simulink model "WhiteBlancing_using_difference_of_255"  (R2016a)
settings: Solver=VariableStepAuto  StartTime=0.0  StopTime=10.0  RelTol=1e-3
undefined symbols (not defined in the file): Rec, SDTV
libraries: visionsources x2, visionsinks x2, visionconversions x1
settings Model: Creator=YASARA  LastModifiedBy=YASARA

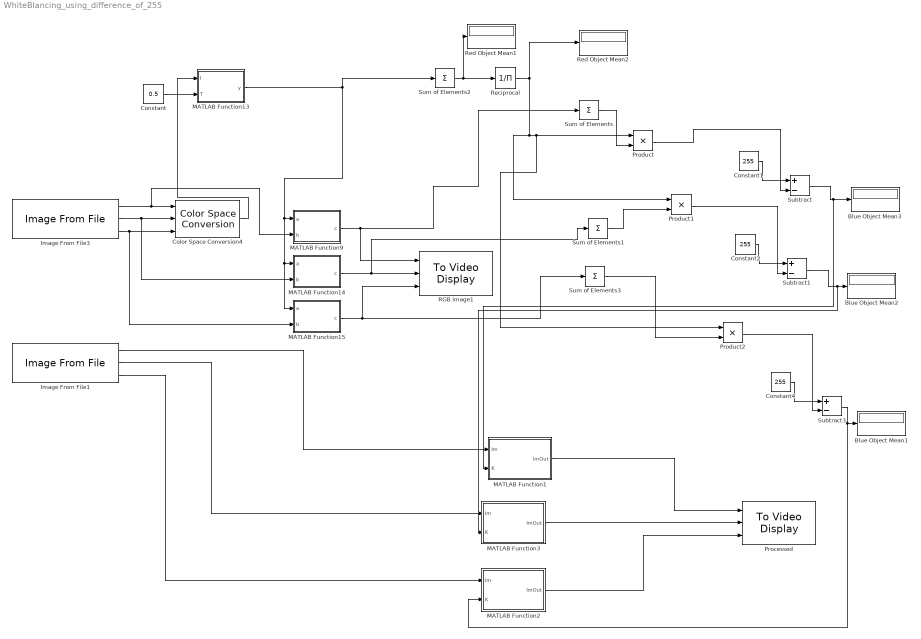
== system WhiteBlancing_using_difference_of_255 ==
  Blue Object Mean1 : Display
  Blue Object Mean2 : Display
  Blue Object Mean3 : Display
  Color Space Conversion4 : visionconversions/Color Space  Conversion  conversion=Obsolete  conversionActive=R'G'B' to intensity  wp_str=D65  rec=Rec. 601 (SDTV)  sys=1125/60/2:1  imagePorts=Separate color signals
  Constant : Constant  Value=0.5  SampleTime=1
  Constant1 : Constant  Value=255
  Constant2 : Constant  Value=255
  Constant4 : Constant  Value=255
  Image From File1 : visionsources/Image From File  Tag=vipblks_nd  FileName=C:\Users\YASARA\Desktop\FRY_Docu\tea\teaxb.jpg  imagePorts=Separate color signals  Ts=1  ImageDataType=uint8  Signed=on  WordLength=16  sdImageDataType=uint(8)  FractionLengthMode=User-defined  FractionLength=15  OutPortLabels=R|G|B
  Image From File3 : visionsources/Image From File  Tag=vipblks_nd  FileName=C:\Users\YASARA\Desktop\FRY_Docu\tea\teaxb.jpg  imagePorts=Separate color signals  Ts=1  ImageDataType=single  Signed=on  WordLength=16  sdImageDataType=uint(8)  FractionLengthMode=User-defined  FractionLength=15  OutPortLabels=R|G|B
  MATLAB Function1 : MATLAB Function  TreatAsAtomicUnit=on
  MATLAB Function13 : MATLAB Function  TreatAsAtomicUnit=on
  MATLAB Function14 : MATLAB Function  TreatAsAtomicUnit=on
  MATLAB Function15 : MATLAB Function  TreatAsAtomicUnit=on
  MATLAB Function2 : MATLAB Function  TreatAsAtomicUnit=on
  MATLAB Function3 : MATLAB Function  TreatAsAtomicUnit=on
  MATLAB Function9 : MATLAB Function  TreatAsAtomicUnit=on
  Processed : visionsinks/To Video Display  windowSizeMode=Normal  openAtMdlStart=on  fullScreen=off  videoWindowX=252  videoWindowY=213  saveWindowSize=off  videoWindowWidth=512  videoWindowHeight=384  inputColorFormat=RGB  inputType=Obsolete  imagePorts=Separate color signals  OutputDevice=On-screen video monitor  dataOrg=Column-major  isWindowOpen=off
  Product : Product  OutDataTypeStr=uint8
  Product1 : Product  OutDataTypeStr=uint8
  Product2 : Product  OutDataTypeStr=uint8
  RGB image1 : visionsinks/To Video Display  windowSizeMode=Normal  openAtMdlStart=on  fullScreen=off  videoWindowX=252  videoWindowY=213  saveWindowSize=off  videoWindowWidth=512  videoWindowHeight=384  inputColorFormat=RGB  inputType=Obsolete  imagePorts=Separate color signals  OutputDevice=On-screen video monitor  dataOrg=Column-major  isWindowOpen=off
  Reciprocal : Product  Inputs=/  OutDataTypeStr=double  SaturateOnIntegerOverflow=on  RndMeth=Zero
  Red Object Mean1 : Display
  Red Object Mean2 : Display
  Subtract : Sum  Inputs=+-
  Subtract1 : Sum  Inputs=+-
  Subtract3 : Sum  Inputs=+-
  Sum of Elements : Sum  Inputs=+
  Sum of Elements1 : Sum  Inputs=+
  Sum of Elements2 : Sum  Inputs=+  AccumDataTypeStr=uint8  OutDataTypeStr=uint8
  Sum of Elements3 : Sum  Inputs=+
  wires:
  Color Space Conversion4/1 -> MATLAB Function13/1(I)
  Sum of Elements/1 -> Product/2
  MATLAB Function9/1(c) -> RGB image1/1, Sum of Elements/1
  MATLAB Function14/1(c) -> RGB image1/2, Sum of Elements1/1
  Sum of Elements3/1 -> Product2/2
  MATLAB Function15/1(c) -> Sum of Elements3/1, RGB image1/3
  Constant/1 -> MATLAB Function13/2(T)
  Sum of Elements2/1 -> Red Object Mean1/1, Reciprocal/1
  Sum of Elements1/1 -> Product1/2
  Reciprocal/1 -> Red Object Mean2/1, Product1/1, Product2/1, Product/1
  MATLAB Function13/1(y) -> MATLAB Function15/1(a), MATLAB Function14/1(a), MATLAB Function9/1(a), Sum of Elements2/1
  Image From File3/1 -> MATLAB Function9/2(b), Color Space Conversion4/1
  Image From File3/2 -> MATLAB Function14/2(b), Color Space Conversion4/2
  Image From File3/3 -> MATLAB Function15/2(b), Color Space Conversion4/3
  Constant1/1 -> Subtract/1
  Product/1 -> Subtract/2
  Constant2/1 -> Subtract1/1
  Product1/1 -> Subtract1/2
  Constant4/1 -> Subtract3/1
  Product2/1 -> Subtract3/2
  Image From File1/1 -> MATLAB Function1/1(Im)
  Image From File1/2 -> MATLAB Function3/1(Im)
  Image From File1/3 -> MATLAB Function2/1(Im)
  MATLAB Function1/1(ImOut) -> Processed/1
  MATLAB Function3/1(ImOut) -> Processed/2
  MATLAB Function2/1(ImOut) -> Processed/3
  Subtract/1 -> MATLAB Function1/2(K), Blue Object Mean3/1
  Subtract1/1 -> MATLAB Function3/2(K), Blue Object Mean2/1
  Subtract3/1 -> MATLAB Function2/2(K), Blue Object Mean1/1

== matlab function WhiteBlancing_using_difference_of_255/MATLAB Function1 ==
  data: Im input; K input; ImOut output
function ImOut = fcn(Im,K)
%#codegen
coder.extrinsic('imadd');
ImOut =Im;
ImOut=imadd(Im,K);
return

== matlab function WhiteBlancing_using_difference_of_255/MATLAB Function2 ==
  data: Im input; K input; ImOut output
function ImOut = fcn(Im,K)
%#codegen
coder.extrinsic('imadd');
ImOut =Im;
ImOut=imadd(Im,K);
return

== matlab function WhiteBlancing_using_difference_of_255/MATLAB Function3 ==
  data: Im input; K input; ImOut output
function ImOut = fcn(Im,K)
%#codegen
coder.extrinsic('imadd');
ImOut =Im;
ImOut=imadd(Im,K);
return

== matlab function WhiteBlancing_using_difference_of_255/MATLAB Function14 ==
  data: a input; b input; c output
function c = fcn(a,b)
%#codegen
c=a.*b;
return

== matlab function WhiteBlancing_using_difference_of_255/MATLAB Function13 ==
  data: I input; y output; T input
function y = fcn(I,T)
%#codegen
BW = imbinarize(I,T);
y = BW;

== matlab function WhiteBlancing_using_difference_of_255/MATLAB Function15 ==
  data: a input; b input; c output
function c = fcn(a,b)
%#codegen
c=a.*b;
return

== matlab function WhiteBlancing_using_difference_of_255/MATLAB Function9 ==
  data: a input; b input; c output
function c = fcn(a,b)
%#codegen
c=a.*b;
return
